simulink model "psbtransformer"  (Simulink 6.0)
settings: Solver=ode15s  SolverMode=SingleTasking  StartTime=0.0  StopTime=0.1  RelTol=1e-3  AbsTol=1e-6
libraries: powerlib2 x14
settings Model: Creator=patrice  LastModifiedBy=batserve  ExtModeTrigMode=oneshot  ExtModeArmWhenConnect=off  ExtModeAutoUpdateStatusClock=off
settings DataIOCC: LimitDataPoints=off
settings OptimizationCC: BooleanDataType=off
settings DebuggingCC: SolverPrmCheckMsg=none
settings HardwareCC: TargetUnknown=on
settings RTWCC: TemplateMakefile=grt_unix.tmf

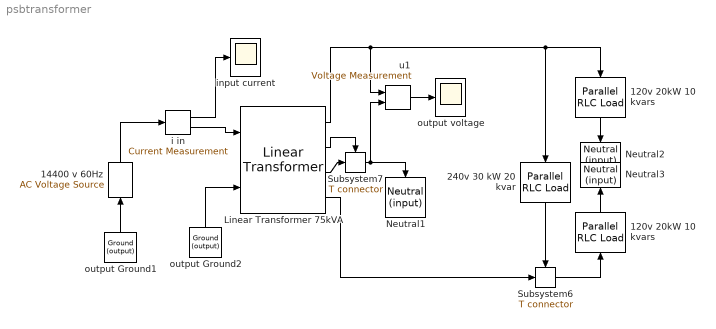
== system psbtransformer ==
  120v 20kW 10 kvars : powerlib2/Elements/Parallel RLC Load  Tag=PoWeRsYsTeMbLoCk  Orientation=down  a=120  b=60  c=20e3  d=10e3  e=0  mesure=None  PSBOutputType=1
  "120v 20kW 10 kvars " : powerlib2/Elements/Parallel RLC Load  Tag=PoWeRsYsTeMbLoCk  Orientation=up  a=120  b=60  c=20e3  d=10e3  e=0  mesure=None  PSBOutputType=1
  14400 v 60Hz : powerlib2/Electrical Sources/AC Voltage Source  Tag=PoWeRsYsTeMbLoCk  Orientation=up  A=14400*sqrt(2)  P=0  F=60  stime=0  mesure=None  PSBOutputType=1
  240v 30 kW 20 kvar : powerlib2/Elements/Parallel RLC Load  Tag=PoWeRsYsTeMbLoCk  Orientation=down  a=240  b=60  c=30e3  d=0  e=20e3  mesure=None  PSBOutputType=1
  "Linear Transformer 75kVA " : powerlib2/Elements/Linear Transformer  Tag=PoWeRsYsTeMbLoCk  a=[75e3,60]  b=[14.4e3 0.01,0.03]  c=[120,0.02,0]  d=[120,0.02,0]  e=[50,50]  mesure=None  PSBOutputType=1111
  Neutral1 : powerlib2/Connectors/Neutral (input)  Tag=PoWeRsYsTeMbLoCk  Orientation=down  no=50
  Neutral2 : powerlib2/Connectors/Neutral (input)  Tag=PoWeRsYsTeMbLoCk  Orientation=down  no=50
  Neutral3 : powerlib2/Connectors/Neutral (input)  Tag=PoWeRsYsTeMbLoCk  Orientation=up  no=50
  Subsystem6 : powerlib2/Connectors/T connector  Tag=PoWeRsYsTeMbLoCk  PSBOutputType=1
  Subsystem7 : powerlib2/Connectors/T connector  Tag=PoWeRsYsTeMbLoCk  PSBOutputType=1
  i in : powerlib2/Measurements/Current Measurement  Tag=PoWeRsYsTeMmEaSuReMeNt  PSBOutputType=01  PSBequivalent=0
  input current : Scope
      settings: DeleteFcn=simscope BlockIsBeingDestroyed  PostSaveFcn=simscope Save  TickLabels=on  TimeRange=0.1  YMin=-10  YMax=10  DataFormat=Array
  output voltage : Scope
      settings: DeleteFcn=simscope BlockIsBeingDestroyed  PostSaveFcn=simscope Save  TickLabels=on  TimeRange=0.1  YMin=-200  YMax=200  DataFormat=Array
  output Ground1 : powerlib2/Connectors/Ground (output)  Tag=PoWeRsYsTeMbLoCk  Orientation=up  PSBOutputType=1
  output Ground2 : powerlib2/Connectors/Ground (output)  Tag=PoWeRsYsTeMbLoCk  Orientation=up  PSBOutputType=1
  u1 : powerlib2/Measurements/Voltage Measurement  Tag=PoWeRsYsTeMmEaSuReMeNt  PSBOutputType=0  PSBequivalent=1
  wires:
  output Ground2/1 -> "Linear Transformer 75kVA "/2
  output Ground1/1 -> 14400 v 60Hz/1
  240v 30 kW 20 kvar/1 -> Subsystem6/Enable
  Subsystem6/1 -> "120v 20kW 10 kvars "/1
  "120v 20kW 10 kvars "/1 -> Neutral3/1
  120v 20kW 10 kvars/1 -> Neutral2/1
  14400 v 60Hz/1 -> i in/1
  i in/2 -> "Linear Transformer 75kVA "/1
  "Linear Transformer 75kVA "/4 -> Subsystem6/1
  "Linear Transformer 75kVA "/3 -> Subsystem7/1
  "Linear Transformer 75kVA "/2 -> Subsystem7/Enable
  Subsystem7/1 -> Neutral1/1, u1/2
  "Linear Transformer 75kVA "/1 -> 240v 30 kW 20 kvar/1, 120v 20kW 10 kvars/1, u1/1
  i in/1 -> input current/1
  u1/1 -> output voltage/1
